simulink model "fangzhen_1"  (R2018b)
settings: Solver=FixedStepAuto  StartTime=0.0  StopTime=40  FixedStep=0.01  RelTol=1e-3
settings Model: Creator=ltiger  LastModifiedBy=QJ-
settings SFSimCC: SimUseLocalCustomCode=off
settings RTWCC: RTWUseLocalCustomCode=off
settings CodeAppCC: StateflowObjectComments=on

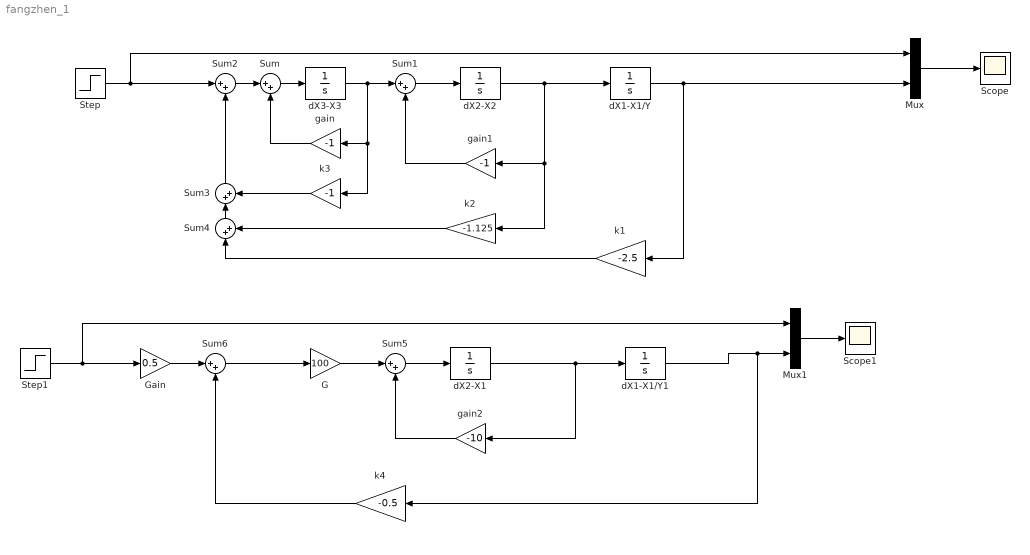
== system fangzhen_1 ==
  G : Gain  Gain=100
  Gain : Gain  Gain=0.5
  Mux : Mux  Inputs=2
  Mux1 : Mux  Inputs=2
  Scope : Scope
  Scope1 : Scope
  Step : Step  SampleTime=0
  Step1 : Step  After=2  SampleTime=0
  Sum{,1..6} (7 alike) : Sum  Inputs=|++
  dX1-X1/Y : TransferFcn  Denominator=[1 0]
  dX1-X1/Y1 : TransferFcn  Denominator=[1 0]
  dX2-X1 : TransferFcn  Denominator=[1 0]
  dX2-X2 : TransferFcn  Denominator=[1 0]
  dX3-X3 : TransferFcn  Denominator=[1 0]
  gain : Gain  Gain=-1
  gain1 : Gain  Gain=-1
  gain2 : Gain  Gain=-10
  k1 : Gain  Gain=-2.5
  k2 : Gain  Gain=-1.125
  k3 : Gain  Gain=-1
  k4 : Gain  Gain=-0.5
  wires:
  Sum/1 -> dX3-X3/1
  Step/1 -> Sum2/1, Mux/1
  gain/1 -> Sum/2
  dX3-X3/1 -> k3/1, gain/1, Sum1/1
  gain1/1 -> Sum1/2
  Sum1/1 -> dX2-X2/1
  dX2-X2/1 -> k2/1, gain1/1, dX1-X1/Y/1
  Mux/1 -> Scope/1
  dX1-X1/Y/1 -> k1/1, Mux/2
  Sum2/1 -> Sum/1
  k3/1 -> Sum3/2
  Sum3/1 -> Sum2/2
  Sum4/1 -> Sum3/1
  k2/1 -> Sum4/2
  k1/1 -> Sum4/1
  dX2-X1/1 -> gain2/1, dX1-X1/Y1/1
  Sum5/1 -> dX2-X1/1
  gain2/1 -> Sum5/2
  G/1 -> Sum5/1
  Sum6/1 -> G/1
  dX1-X1/Y1/1 -> k4/1, Mux1/2
  Mux1/1 -> Scope1/1
  k4/1 -> Sum6/2
  Step1/1 -> Gain/1, Mux1/1
  Gain/1 -> Sum6/1
